simulink model "determine_force_mass_inertia"  (R2020b)
settings: Solver=VariableStepAuto  StartTime=0.0  StopTime=10.0  RelTol=1e-3
values from neighbouring files (symbols this model uses):
  inertia = diag([Ixx, Iyy, Izz])    [iris_quadcopter_specs.m]
settings Model: Creator=sid  LastModifiedBy=sid

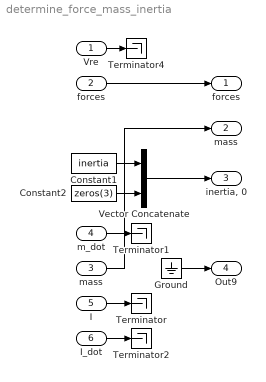
== system determine_force_mass_inertia ==
  Vre : Inport
  forces : Inport  Port=2
  "mass " : Inport  Port=3
  m_dot : Inport  Port=4  OutDataTypeStr=double
  I : Inport  Port=5  OutDataTypeStr=double
  I_dot : Inport  Port=6  OutDataTypeStr=double
  Constant1 : Constant  Value=inertia  OutDataTypeStr=Inherit: Inherit via back propagation
  Constant2 : Constant  Value=zeros(3)
  Ground : Ground
  Terminator{,1..2,4} (4 alike) : Terminator
  Vector Concatenate : Concatenate  Mode=Multidimensional array
  "forces " : Outport  VectorParamsAs1DForOutWhenUnconnected=off
  mass : Outport  Port=2  VectorParamsAs1DForOutWhenUnconnected=off
  "inertia, 0" : Outport  Port=3  VectorParamsAs1DForOutWhenUnconnected=off
  Out9 : Outport  Port=4  VectorParamsAs1DForOutWhenUnconnected=off
  wires:
  Ground/1 -> Out9/1
  "mass "/1 -> mass/1
  Constant2/1 -> Vector Concatenate/2
  I_dot/1 -> Terminator2/1
  Constant1/1 -> Vector Concatenate/1
  forces/1 -> "forces "/1
  m_dot/1 -> Terminator1/1
  Vector Concatenate/1 -> "inertia, 0"/1
  I/1 -> Terminator/1
  Vre/1 -> Terminator4/1
